simulink model "ModulacionAM"  (R2019a)
settings: Solver=VariableStepAuto  StartTime=0.0  StopTime=4  RelTol=1e-3
settings Model: NumberOfSteps=3  Creator=JORGE  LastModifiedBy=JORGE

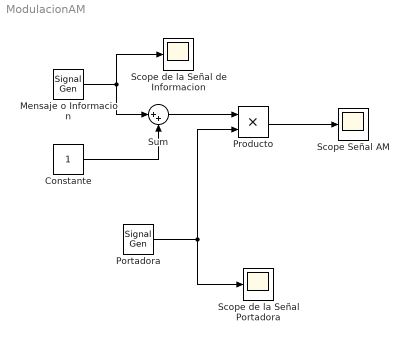
== system ModulacionAM ==
  "    \t   Sum" : Sum  Inputs=|++
  "Constante " : Constant
  Mensaje o Informacion : SignalGenerator
  "Portadora " : SignalGenerator  Frequency=20
  "Producto " : Product
  Scope Señal AM : Scope
  "Scope de la Señal de Informacion " : Scope
  Scope de la Señal Portadora : Scope
  wires:
  Mensaje o Informacion/1 -> "Scope de la Señal de Informacion "/1, "    \t   Sum"/1
  "Constante "/1 -> "    \t   Sum"/2
  "    \t   Sum"/1 -> "Producto "/1
  "Portadora "/1 -> Scope de la Señal Portadora/1, "Producto "/2
  "Producto "/1 -> Scope Señal AM/1
